simulink library "universalSpoolingController_ul"  (R2022a)
settings: Solver=VariableStepAuto  StartTime=0.0  StopTime=10.0  RelTol=1e-3
undefined symbols (not defined in the file or in its folder): DiscIntNeverNeededParam, fltCtrl, pathCtrl, runningAvg, runningAvg_ul, SPOOLINGCONTROLLER
libraries: simulink x5, dspsigops x1, stopwatch_ul x1
settings Model: Creator=James Reed  LastModifiedBy=lhill8
settings SolverCC: AlgebraicLoopSolver=TrustRegion
settings DebuggingCC: UnconnectedInputMsg=warning  UnconnectedOutputMsg=warning  UnconnectedLineMsg=warning  SFMachineParentedDataDiag=warning  ArithmeticOperatorsInVariantConditions=warning
settings SFSimCC: CustomCodeUndefinedFunction=UseInterfaceOnly

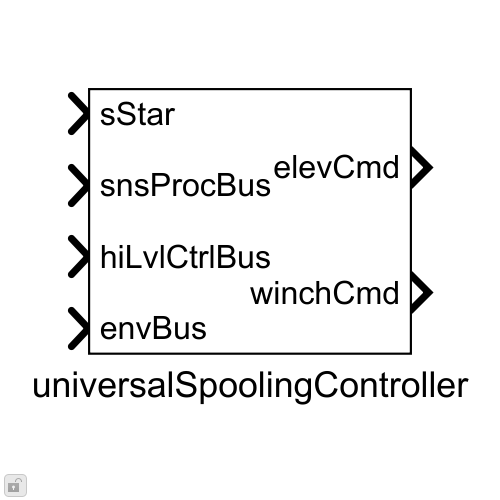
[thumbnail: Simulink's stored preview of the top-level diagram]
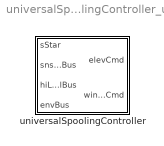
== system universalSpoolingController_ul ==
  universalSpoolingController : Subsystem  VariantControl=strcmpi(SPOOLINGCONTROLLER,'universalSpoolingController')  mask{reelInDefl=fltCtrl.elevatorReelInDef.Value, reelOutDefl=0, ctrlVecInit=fltCtrl.initCtrlVec.Value, spdVecInit=fltCtrl.initSpdVec.Value, firstSpoolLap=fltCtrl.firstSpoolLap.Value}
      mask prompts: reelInDefl "Reel In Elevator Deflection [deg]"; reelOutDefl "Reel Out Elevator Deflection [deg]"; ctrlVecInit "Init ctrlVec (defined in Matlab Fcns)"; spdVecInit "Init spdVec (defined in Matlab Fcns)"; firstSpoolLap "First Lap to Begin Spooling"
      mask TypeOptions reelInDefl: ReelInElevDefl1/Value
      mask TypeOptions reelOutDefl: ReelOutElevDefl1/Value

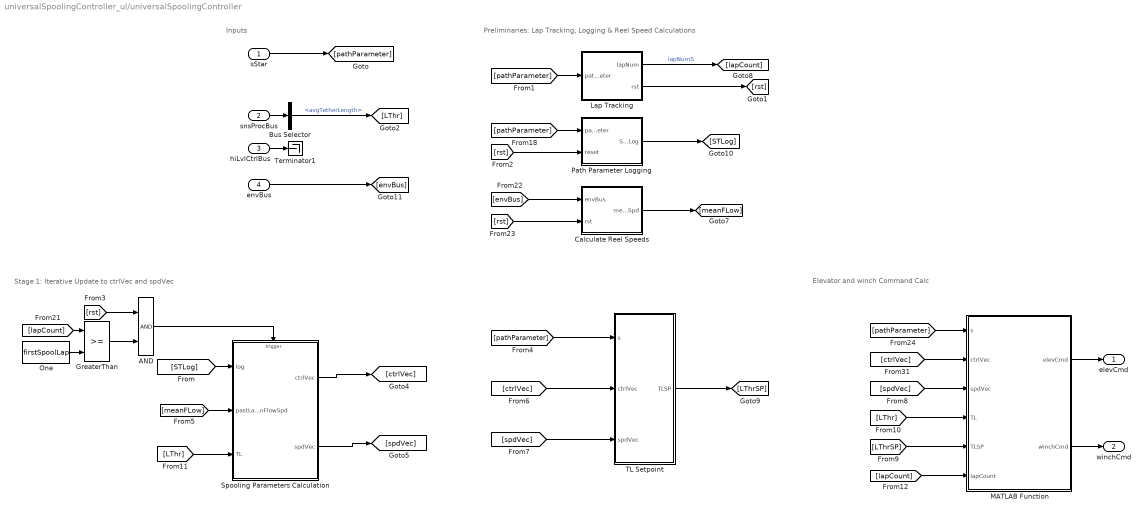
== system universalSpoolingController_ul/universalSpoolingController ==
  note: Elevator and winch Command Calc
  note: Stage 1: Iterative Update to ctrlVec and spdVec
  note: Inputs
  note: Preliminaries: Lap Tracking, Logging & Reel Speed Calculations
  "sStar " : Inport
  snsProcBus : Inport  Port=2  OutDataTypeStr=Bus: sensorsProcessingBus
  hiLvlCtrlBus : Inport  Port=3  OutDataTypeStr=Bus: hiLvlCtrlBus
  envBus : Inport  Port=4  OutDataTypeStr=Bus: envBus
  AND : Logic  AllPortsSameDT=off  OutDataTypeStr=boolean
  Bus Selector : BusSelector  OutputSignals=avgTetherLength
  Calculate Reel Speeds : Subsystem
  GreaterThan : RelationalOperator  OutDataTypeStr=boolean  RndMeth=Simplest  InputSameDT=off
  Lap Tracking : Subsystem
  MATLAB Function : MATLAB Function  TreatAsAtomicUnit=on  mask{elevDeflIn=pathCtrl.elevatorReelInDef.Value, firstSpoolLap=pathCtrl.firstSpoolLap.Value}
      mask prompts: elevDeflIn "elevator Deflection In"; firstSpoolLap "Lap to begin spooling"
  One : Constant  Value=firstSpoolLap  OutDataTypeStr=Inherit: Inherit via back propagation
  Path Parameter Logging : Subsystem
  Spooling Parameters Calculation : Subsystem  TreatAsAtomicUnit=on
  TL Setpoint : MATLAB Function  TreatAsAtomicUnit=on
  Terminator1 : Terminator
  elevCmd : Outport  VectorParamsAs1DForOutWhenUnconnected=off
  winchCmd : Outport  Port=2  VectorParamsAs1DForOutWhenUnconnected=off
  wires:
  AND/1 -> Spooling Parameters Calculation/Trigger
  GreaterThan/1 -> AND/2
  [rst] -> AND/1
  One/1 -> GreaterThan/2
  [lapCount] -> GreaterThan/1
  hiLvlCtrlBus/1 -> Terminator1/1
  "sStar "/1 -> [pathParameter]
  Bus Selector/1 -> [LThr]  "<avgTetherLength>"
  Spooling Parameters Calculation/1(ctrlVec) -> [ctrlVec]
  Spooling Parameters Calculation/2(spdVec) -> [spdVec]
  [pathParameter] -> Path Parameter Logging/1(pathParameter)
  [rst] -> Path Parameter Logging/2(reset)
  Path Parameter Logging/1(SVsTLog) -> [STLog]
  [STLog] -> Spooling Parameters Calculation/1(log)
  envBus/1 -> [envBus]
  [envBus] -> Calculate Reel Speeds/1(envBus)
  Calculate Reel Speeds/1(meanFlowSpd) -> [meanFLow]
  [rst] -> Calculate Reel Speeds/2(rst)
  [pathParameter] -> Lap Tracking/1(pathParameter)
  Lap Tracking/1(lapNum) -> [lapCount]  "lapNumS"
  Lap Tracking/2(rst) -> [rst]
  TL Setpoint/1(TLSP) -> [LThrSP]
  [pathParameter] -> MATLAB Function/1(s)
  snsProcBus/1 -> Bus Selector/1
  [ctrlVec] -> MATLAB Function/2(ctrlVec)
  [meanFLow] -> Spooling Parameters Calculation/2(pastLapMeanFlowSpd)
  [spdVec] -> TL Setpoint/3(spdVec)
  [pathParameter] -> TL Setpoint/1(s)
  [ctrlVec] -> TL Setpoint/2(ctrlVec)
  [spdVec] -> MATLAB Function/3(spdVec)
  [LThrSP] -> MATLAB Function/5(TLSP)
  [LThr] -> MATLAB Function/4(TL)
  MATLAB Function/1(elevCmd) -> elevCmd/1
  MATLAB Function/2(winchCmd) -> winchCmd/1
  [LThr] -> Spooling Parameters Calculation/3(TL)
  [lapCount] -> MATLAB Function/6(lapCount)

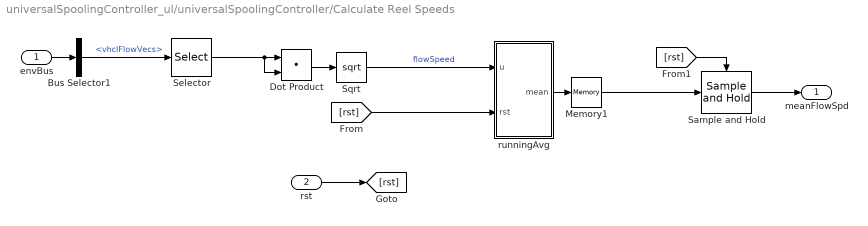
== system universalSpoolingController_ul/universalSpoolingController/Calculate Reel Speeds ==
  envBus : Inport
  rst : Inport  Port=2
  Bus Selector1 : BusSelector  OutputSignals=vhclFlowVecs
  Dot Product : DotProduct  OutDataTypeStr=Inherit: Inherit via internal rule
  Memory1 : Memory
  Sample and Hold : dspsigops/Sample and Hold  trig=Rising edge  initCond=0  latchinput=off
  Selector : Selector  NumberOfDimensions=2  InputPortWidth=3  IndexOptions=Select all,Index vector (dialog)  Indices=[1 3],5  OutputSizes=1,1
  Sqrt : Sqrt
  runningAvg : Subsystem  AncestorBlock=runningAvg_ul/runningAvg
  meanFlowSpd : Outport  VectorParamsAs1DForOutWhenUnconnected=off
  wires:
  Sample and Hold/1 -> meanFlowSpd/1
  rst/1 -> [rst]
  Bus Selector1/1 -> Selector/1  "<vhclFlowVecs>"
  runningAvg/1(mean) -> Memory1/1
  Sqrt/1 -> runningAvg/1(u)  "flowSpeed"
  envBus/1 -> Bus Selector1/1
  Memory1/1 -> Sample and Hold/1
  [rst] -> runningAvg/2(rst)
  [rst] -> Sample and Hold/Trigger
  Selector/1 -> Dot Product/2, Dot Product/1
  Dot Product/1 -> Sqrt/1

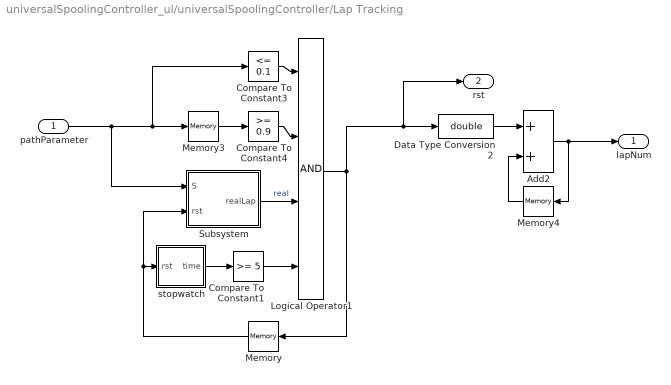
== system universalSpoolingController_ul/universalSpoolingController/Lap Tracking ==
  pathParameter : Inport
  Add2 : Sum
  Compare To Constant1 : simulink/Logic and Bit Operations/Compare To Constant  relop=>=  const=5  OutDataTypeStr=boolean
  Compare To Constant3 : simulink/Logic and Bit Operations/Compare To Constant  relop=<=  const=0.1  OutDataTypeStr=boolean
  Compare To Constant4 : simulink/Logic and Bit Operations/Compare To Constant  relop=>=  const=0.9  OutDataTypeStr=boolean
  Data Type Conversion2 : DataTypeConversion  OutDataTypeStr=double  SaturateOnIntegerOverflow=off  RndMeth=Floor
  Logical Operator1 : Logic  Inputs=4  AllPortsSameDT=off  OutDataTypeStr=boolean
  Memory : Memory  InitialCondition=false
  Memory3 : Memory
  Memory4 : Memory
  Subsystem : Subsystem
  stopwatch : Subsystem  AncestorBlock=stopwatch_ul/stopwatch
  lapNum : Outport  VectorParamsAs1DForOutWhenUnconnected=off
  rst : Outport  Port=2  VectorParamsAs1DForOutWhenUnconnected=off
  wires:
  Compare To Constant3/1 -> Logical Operator1/1
  Data Type Conversion2/1 -> Add2/1
  Logical Operator1/1 -> rst/1, Data Type Conversion2/1, Memory/1
  Memory4/1 -> Add2/2
  Add2/1 -> lapNum/1, Memory4/1
  Compare To Constant4/1 -> Logical Operator1/2
  pathParameter/1 -> Subsystem/1(S), Compare To Constant3/1, Memory3/1
  stopwatch/1(time) -> Compare To Constant1/1
  Memory/1 -> Subsystem/2(rst), stopwatch/1(rst)
  Compare To Constant1/1 -> Logical Operator1/4
  Subsystem/1(realLap) -> Logical Operator1/3  "real"
  Memory3/1 -> Compare To Constant4/1

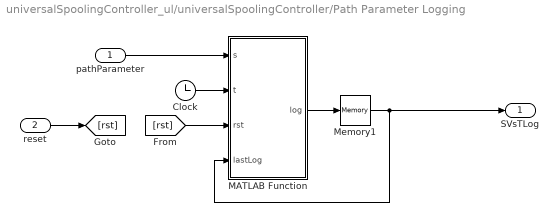
== system universalSpoolingController_ul/universalSpoolingController/Path Parameter Logging ==
  pathParameter : Inport
  reset : Inport  Port=2
  Clock : Clock
  MATLAB Function : MATLAB Function  TreatAsAtomicUnit=on
  Memory1 : Memory  InitialCondition=zeros(1000,2)
  SVsTLog : Outport  VectorParamsAs1DForOutWhenUnconnected=off
  wires:
  MATLAB Function/1(log) -> Memory1/1
  reset/1 -> [rst]
  pathParameter/1 -> MATLAB Function/1(s)
  Clock/1 -> MATLAB Function/2(t)
  Memory1/1 -> SVsTLog/1, MATLAB Function/4(lastLog)
  [rst] -> MATLAB Function/3(rst)

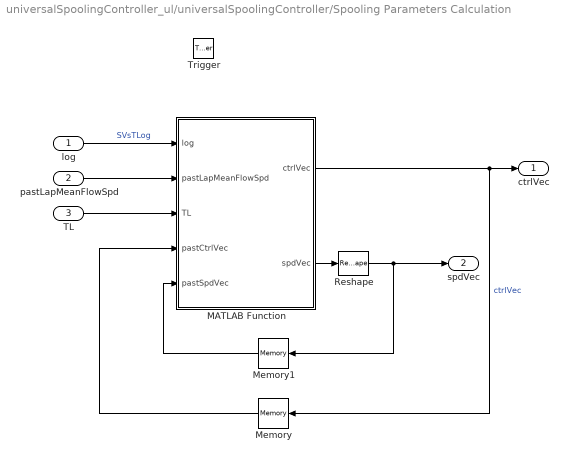
== system universalSpoolingController_ul/universalSpoolingController/Spooling Parameters Calculation ==
  log : Inport
  pastLapMeanFlowSpd : Inport  Port=2
  TL : Inport  Port=3
  Trigger : TriggerPort  VariantControl=Variant
  MATLAB Function : MATLAB Function  TreatAsAtomicUnit=on  mask{intraDrift=fltCtrl.intraDrift.Value}
      mask prompts: intraDrift "Intra-Cycle Net Spooling per lap"
  Memory : Memory  InitialCondition=ctrlVecInit  InheritSampleTime=on
  Memory1 : Memory  InitialCondition=spdVecInit  InheritSampleTime=on
  Reshape : Reshape
  ctrlVec : Outport  InitialOutput=ctrlVecInit  VectorParamsAs1DForOutWhenUnconnected=off
  spdVec : Outport  Port=2  InitialOutput=spdVecInit  VectorParamsAs1DForOutWhenUnconnected=off
  wires:
  log/1 -> MATLAB Function/1(log)  "SVsTLog"
  Memory/1 -> MATLAB Function/4(pastCtrlVec)
  pastLapMeanFlowSpd/1 -> MATLAB Function/2(pastLapMeanFlowSpd)
  MATLAB Function/1(ctrlVec) -> Memory/1, ctrlVec/1  "ctrlVec"
  TL/1 -> MATLAB Function/3(TL)
  MATLAB Function/2(spdVec) -> Reshape/1
  Memory1/1 -> MATLAB Function/5(pastSpdVec)
  Reshape/1 -> Memory1/1, spdVec/1

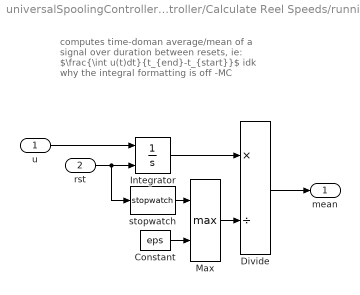
== system universalSpoolingController_ul/universalSpoolingController/Calculate Reel Speeds/runningAvg ==
  note: computes time-doman average/mean of a
      | signal over duration between resets, ie:
      | $\frac{\int u(t)dt}{t_{end}-t_{start}}$
      | idk why the integral formatting is off -MC
  u : Inport
  rst : Inport  Port=2
  Constant : Constant  Value=eps
  Divide : Product  Inputs=*/
  Integrator : Integrator  ExternalReset=rising
  Max : MinMax  Function=max  Inputs=2
  stopwatch : stopwatch_ul/stopwatch  SystemSampleTime=-1  VariantActivationTime=update diagram  Latency=0  AutoFrameSizeCalculation=off
  mean : Outport  VectorParamsAs1DForOutWhenUnconnected=off
  wires:
  rst/1 -> Integrator/2, stopwatch/1
  Max/1 -> Divide/2
  Constant/1 -> Max/2
  Divide/1 -> mean/1
  stopwatch/1 -> Max/1
  u/1 -> Integrator/1
  Integrator/1 -> Divide/1

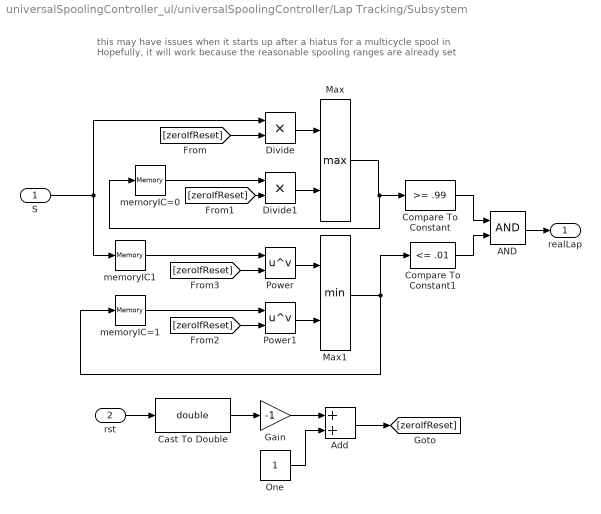
== system universalSpoolingController_ul/universalSpoolingController/Lap Tracking/Subsystem ==
  note: this may have issues when it starts up after a hiatus for a multicycle spool in
      | Hopefully, it will work because the reasonable spooling ranges are already set
  S : Inport
  rst : Inport  Port=2
  AND : Logic  AllPortsSameDT=off  OutDataTypeStr=boolean
  Add : Sum
  Cast To Double : DataTypeConversion  OutDataTypeStr=double  SaturateOnIntegerOverflow=off  RndMeth=Floor
  Compare To Constant : simulink/Logic and Bit Operations/Compare To Constant  relop=>=  const=.99  OutDataTypeStr=boolean
  Compare To Constant1 : simulink/Logic and Bit Operations/Compare To Constant  relop=<=  const=.01  OutDataTypeStr=boolean
  Divide : Product  Inputs=**
  Divide1 : Product  Inputs=**
  Gain : Gain  Gain=-1
  Max : MinMax  Function=max  Inputs=2
  Max1 : MinMax  Inputs=2
  One : Constant  OutDataTypeStr=Inherit: Inherit via back propagation
  Power : Math  Operator=pow
  Power1 : Math  Operator=pow
  memoryIC1 : Memory  InitialCondition=1
  memoryIC=0 : Memory
  memoryIC=1 : Memory  InitialCondition=1
  realLap : Outport
  wires:
  Max1/1 -> Compare To Constant1/1, memoryIC=1/1
  rst/1 -> Cast To Double/1
  S/1 -> Divide/1, memoryIC1/1
  Gain/1 -> Add/1
  Add/1 -> [zeroIfReset]
  One/1 -> Add/2
  Divide/1 -> Max/1
  Max/1 -> memoryIC=0/1, Compare To Constant/1
  Power/1 -> Max1/1
  Power1/1 -> Max1/2
  Cast To Double/1 -> Gain/1
  Compare To Constant/1 -> AND/1
  Compare To Constant1/1 -> AND/2
  AND/1 -> realLap/1
  [zeroIfReset] -> Divide/2
  [zeroIfReset] -> Power/2
  [zeroIfReset] -> Divide1/2
  Divide1/1 -> Max/2
  memoryIC=0/1 -> Divide1/1
  [zeroIfReset] -> Power1/2
  memoryIC=1/1 -> Power1/1
  memoryIC1/1 -> Power/1

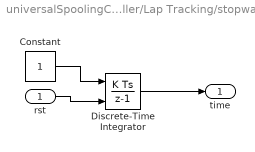
== system universalSpoolingController_ul/universalSpoolingController/Lap Tracking/stopwatch ==
  rst : Inport
  Constant : Constant
  Discrete-Time Integrator : DiscreteIntegrator  ExternalReset=rising  SampleTime=-1  ICPrevOutput=DiscIntNeverNeededParam  ICPrevScaledInput=DiscIntNeverNeededParam
  time : Outport  VectorParamsAs1DForOutWhenUnconnected=off
  wires:
  Constant/1 -> Discrete-Time Integrator/1
  Discrete-Time Integrator/1 -> time/1
  rst/1 -> Discrete-Time Integrator/2

== matlab function universalSpoolingController_ul/universalSpoolingController/MATLAB Function ==
  data: elevCmd output; winchCmd output; s input; ctrlVec input; spdVec input; TL input; TLSP input; lapCount input; elevDeflIn parameter; firstSpoolLap parameter
function [elevCmd, winchCmd] = fcn(s,ctrlVec,spdVec,TL,TLSP,lapCount,elevDeflIn, firstSpoolLap)
    [elevCmd, winchCmd] = combinedCmd(s,ctrlVec,spdVec,TL,TLSP,lapCount,elevDeflIn,firstSpoolLap);
end

== matlab function universalSpoolingController_ul/universalSpoolingController/Path Parameter Logging/MATLAB Function ==
  data: s input; log output; t input; rst input; lastLog input
function log = fcn(s,t,rst,lastLog)
% function that logs the path position and time into a matrix
% [pathPosition,t]
if rst
    lastLog = nan(1000,2);
end
log = lastLog;
idx = min([max([round(s*1000),1]),1000]);
log(idx,1) = s;
log(idx,2) = t;

== matlab function universalSpoolingController_ul/universalSpoolingController/Spooling Parameters Calculation/MATLAB Function ==
  data: log input; pastLapMeanFlowSpd input; TL input; pastCtrlVec input; pastSpdVec input; ctrlVec output; spdVec output; intraDrift parameter
function [ctrlVec,spdVec] = fcn(log,pastLapMeanFlowSpd,TL,pastCtrlVec,pastSpdVec,intraDrift)
    [ctrlVec, spdVec] = combinedCtrl(log,pastLapMeanFlowSpd,TL,pastCtrlVec,pastSpdVec,intraDrift);
end

== matlab function universalSpoolingController_ul/universalSpoolingController/TL Setpoint ==
  data: s input; ctrlVec input; spdVec input; TLSP output
function TLSP = fcn(s,ctrlVec,spdVec) %#ok<*INUSD>
    TLSP = combinedTLSP(s,ctrlVec,spdVec);
end
